simulink model "StateSpace_Modeling"  (R2024a)
settings: Solver=VariableStepAuto  StartTime=0.0  StopTime=10.0  RelTol=1e-3
values from neighbouring files (symbols this model uses):
  br = 0    [parameters.m]
  g = 9.8    [parameters.m]
  Jw = 0    [parameters.m]
  Ke = 0    [parameters.m]
  Kt = 0    [parameters.m]
  La = 0    [parameters.m]
  Lr = 0    [parameters.m]
  Lw = 0    [parameters.m]
  mr = 0    [parameters.m]
  mw = 0    [parameters.m]
  Ra = 0    [parameters.m]
  Va = 0    [parameters.m]
undefined symbols (not defined in the file or in its folder): Jp
settings Model: Creator=Asus1  LastModifiedBy=Asus1

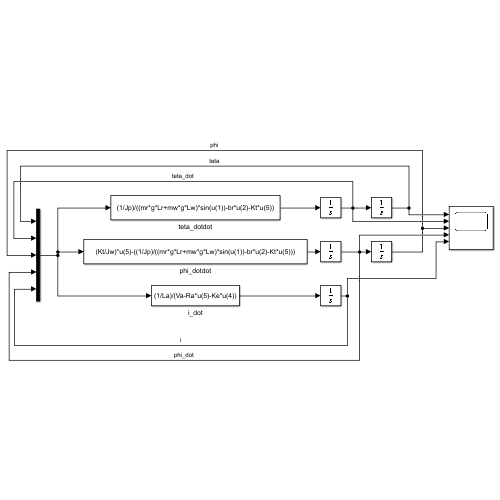
[thumbnail: Simulink's stored preview of the top-level diagram]
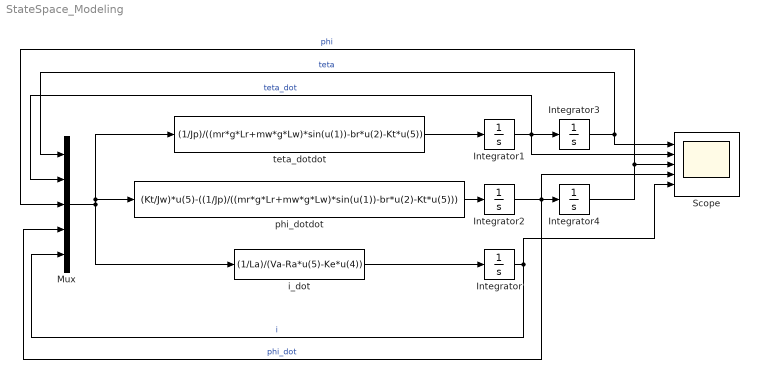
== system StateSpace_Modeling ==
  Integrator{,1..4} (5 alike) : Integrator
  Mux : Mux  Inputs=5
  Scope : Scope  NumInputPorts=5
  i_dot : Fcn  Expr=(1/La)/(Va-Ra*u(5)-Ke*u(4))
  phi_dotdot : Fcn  Expr=(Kt/Jw)*u(5)-((1/Jp)/((mr*g*Lr+mw*g*Lw)*sin(u(1))-br*u(2)-Kt*u(5)))
  teta_dotdot : Fcn  Expr=(1/Jp)/((mr*g*Lr+mw*g*Lw)*sin(u(1))-br*u(2)-Kt*u(5))
  wires:
  i_dot/1 -> Integrator/1
  teta_dotdot/1 -> Integrator1/1
  phi_dotdot/1 -> Integrator2/1
  Mux/1 -> phi_dotdot/1, teta_dotdot/1, i_dot/1
  Integrator2/1 -> Mux/4, Scope/4, Integrator4/1  "phi_dot"
  Integrator1/1 -> Mux/2, Scope/2, Integrator3/1  "teta_dot"
  Integrator3/1 -> Mux/1, Scope/1  "teta"
  Integrator4/1 -> Mux/3, Scope/3  "phi"
  Integrator/1 -> Mux/5, Scope/5  "i"
